simulink model "controlador_traslacion"  (R2019a)
settings: Solver=VariableStepAuto  StartTime=0.0  StopTime=10.0  RelTol=1e-3
values from neighbouring files (symbols this model uses):
  ba_t = 1    [parametros.m]
  Ksa_t = 1    [parametros.m]
  Ksia_t = 1    [parametros.m]
settings Model: Creator=Facundo  LastModifiedBy=Facundo

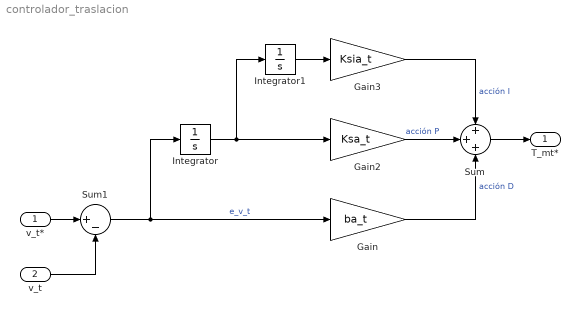
== system controlador_traslacion ==
  v_t* : Inport
  v_t : Inport  Port=2
  Gain : Gain  Gain=ba_t
  Gain2 : Gain  Gain=Ksa_t
  Gain3 : Gain  Gain=Ksia_t
  Integrator : Integrator
  Integrator1 : Integrator
  Sum : Sum  Inputs=+++
  Sum1 : Sum  Inputs=|+-
  T_mt* : Outport
  wires:
  Sum1/1 -> Gain/1, Integrator/1  "e_v_t"
  Integrator/1 -> Gain2/1, Integrator1/1
  Integrator1/1 -> Gain3/1
  Gain2/1 -> Sum/2  "acción P"
  Gain/1 -> Sum/3  "acción D"
  Gain3/1 -> Sum/1  "acción I"
  Sum/1 -> T_mt*/1
  v_t*/1 -> Sum1/1
  v_t/1 -> Sum1/2
